simulink model "linear_with_noise"  (R2017b)
settings: Solver=VariableStepAuto  StartTime=0.0  StopTime=20.0  RelTol=1e-3
libraries: simulink x1
settings Model: Creator=admin  LastModifiedBy=admin

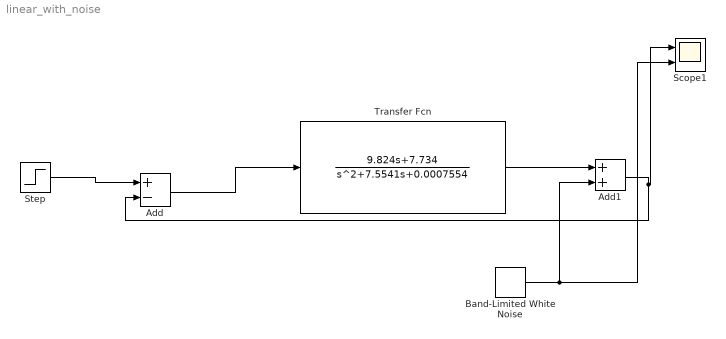
== system linear_with_noise ==
  Add : Sum  Inputs=+-
  Add1 : Sum
  Band-Limited White Noise : simulink/Sources/Band-Limited White Noise  Cov=[0.00000001]  Ts=0.1  seed=[23341]
  Scope1 : Scope  NumInputPorts=2
  Step : Step  After=0.02  SampleTime=0
  Transfer Fcn : TransferFcn  Numerator=[9.824 7.734]  Denominator=[1 7.5541 0.0007554]
  wires:
  Add/1 -> Transfer Fcn/1
  Transfer Fcn/1 -> Add1/1
  Add1/1 -> Scope1/1, Add/2
  Band-Limited White Noise/1 -> Scope1/2, Add1/2
  Step/1 -> Add/1
